simulink model "Question2"  (R2020b)
settings: Solver=FixedStepAuto  StartTime=0.0  StopTime=100.0  FixedStep=0.01  RelTol=1e-3
settings Model: Creator=Murat  LastModifiedBy=Murat

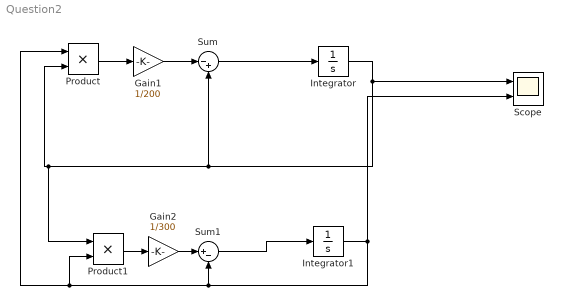
== system Question2 ==
  Gain1 : Gain  Gain=1/200
  Gain2 : Gain  Gain=1/300
  Integrator : Integrator  InitialCondition=400
  Integrator1 : Integrator  InitialCondition=100
  Product : Product
  Product1 : Product
  Scope : Scope  NumInputPorts=2
  Sum : Sum  Inputs=|-+
  Sum1 : Sum  Inputs=|+-
  wires:
  Product/1 -> Gain1/1
  Gain1/1 -> Sum/1
  Sum/1 -> Integrator/1
  Product1/1 -> Gain2/1
  Gain2/1 -> Sum1/1
  Sum1/1 -> Integrator1/1
  Integrator/1 -> Scope/1, Product1/1, Product/2, Sum/2
  Integrator1/1 -> Scope/2, Product/1, Product1/2, Sum1/2
